simulink model "Lab4b"  (R2019b)
settings: Solver=VariableStepAuto  StartTime=0.0  StopTime=10.0  RelTol=1e-3
undefined symbols (not defined in the file): dc
libraries: dspfdesign x2, commfilt2 x1, dspstat3 x1, commsink2 x1, commsynccomp2 x1
settings Model: Creator=z3454314  LastModifiedBy=z3454314

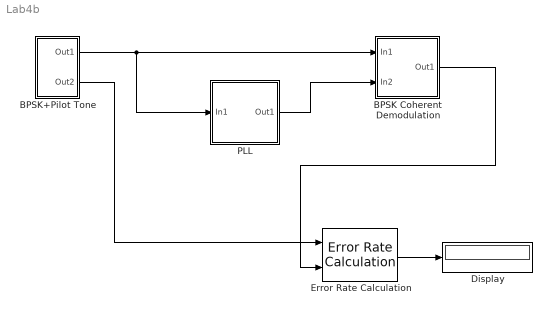
== system Lab4b ==
  BPSK Coherent Demodulation : Subsystem
  BPSK+Pilot Tone : Subsystem
  Display : Display
  Error Rate Calculation : commsink2/Error Rate Calculation  N=2  st_delay=50  cp_mode=Entire frame  subframe=[]  PMode=Port  WsName=ErrorVec  RsMode2=off  stop=off  numErr=100  maxBits=1e6
      settings: SourceProductName=Communications Toolbox
  PLL : Subsystem
  wires:
  Error Rate Calculation/1 -> Display/1
  BPSK+Pilot Tone/2(Out2) -> Error Rate Calculation/1
  BPSK Coherent Demodulation/1(Out1) -> Error Rate Calculation/2
  PLL/1(Out1) -> BPSK Coherent Demodulation/2(In2)
  BPSK+Pilot Tone/1(Out1) -> BPSK Coherent Demodulation/1(In1), PLL/1(In1)

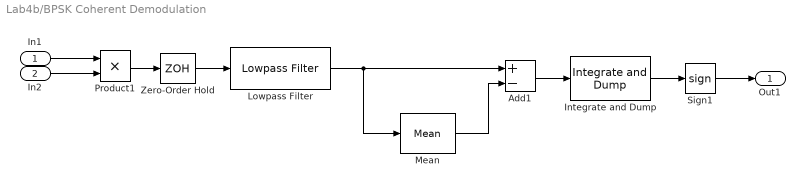
== system Lab4b/BPSK Coherent Demodulation ==
  In1 : Inport
  In2 : Inport  Port=2
  Add1 : Sum  Inputs=+-
  Integrate and Dump : commfilt2/Integrate and Dump  obssamples=1000  offsetsamples=23  nodump=off  roundingMode=Floor  overflowMode=off  outputDataTypeStr=Inherit: Same as accumulator  outputLastDataTypeStr=Inherit: Same as accumulator
      settings: SourceProductName=Communications Toolbox
  Lowpass Filter : dspfdesign/Lowpass Filter  FilterType=FIR  DesignForMinimumOrder=on  FilterOrder=50  PassbandFrequency=6e3  StopbandFrequency=10e3  PassbandRipple=0.1  StopbandAttenuation=80  InheritSampleRate=on  SampleRate=44100  SimulateUsing=Interpreted execution  roundingMode=Floor  coeffsDataTypeStr=fixdt(1,16)
  Mean : dspstat3/Mean  run=on  reset_popup=None  directionMode=Each column  dimension=1  roiEnable=off  roiType=Rectangles  roiPortion=Entire ROI  roiOutput=Individual statistics for each ROI  roiFlag=off  roundingMode=Floor  overflowMode=off  outputDataTypeStr=Inherit: Same as accumulator  outputMin=[]  outputMax=[]  outputLastDataTypeStr=Inherit: Same as accumulator
  Product1 : Product
  Sign1 : Signum
  Zero-Order Hold : ZeroOrderHold  SampleTime=1/500e3
  Out1 : Outport
  wires:
  Mean/1 -> Add1/2
  Zero-Order Hold/1 -> Lowpass Filter/1
  Lowpass Filter/1 -> Mean/1, Add1/1
  In1/1 -> Product1/1
  Integrate and Dump/1 -> Sign1/1
  Product1/1 -> Zero-Order Hold/1
  Sign1/1 -> Out1/1
  Add1/1 -> Integrate and Dump/1
  In2/1 -> Product1/2

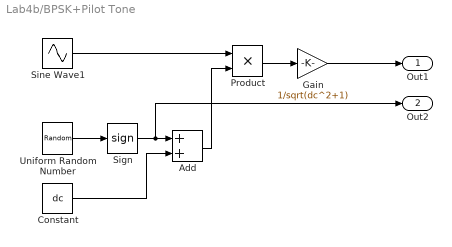
== system Lab4b/BPSK+Pilot Tone ==
  Add : Sum
  Constant : Constant  Value=dc
  Gain : Gain  Gain=1/sqrt(dc^2+1)
  Product : Product
  Sign : Signum
  Sine Wave1 : Sin  Frequency=8020*2*pi  SampleTime=0
  Uniform Random Number : UniformRandomNumber  SampleTime=1/500
  Out1 : Outport
  Out2 : Outport  Port=2
  wires:
  Constant/1 -> Add/2
  Sine Wave1/1 -> Product/1
  Gain/1 -> Out1/1
  Product/1 -> Gain/1
  Sign/1 -> Out2/1, Add/1
  Uniform Random Number/1 -> Sign/1
  Add/1 -> Product/2

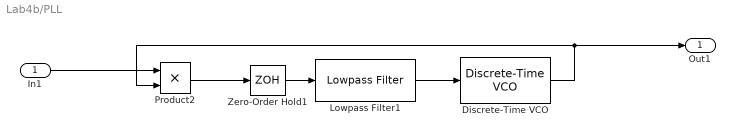
== system Lab4b/PLL ==
  In1 : Inport
  Discrete-Time VCO : commsynccomp2/Discrete-Time VCO  Ac=1  Fc=8000  Kc=100  Ph=0  ts=1/500e3
      settings: SourceProductName=Communications Toolbox  SourceProductBaseCode=CM
  Lowpass Filter1 : dspfdesign/Lowpass Filter  FilterType=FIR  DesignForMinimumOrder=on  FilterOrder=50  PassbandFrequency=5e3  StopbandFrequency=10e3  PassbandRipple=0.1  StopbandAttenuation=80  InheritSampleRate=on  SampleRate=500e3  SimulateUsing=Interpreted execution  roundingMode=Floor  coeffsDataTypeStr=fixdt(1,16)
  Product2 : Product
  Zero-Order Hold1 : ZeroOrderHold  SampleTime=1/500e3
  Out1 : Outport
  wires:
  Product2/1 -> Zero-Order Hold1/1
  Lowpass Filter1/1 -> Discrete-Time VCO/1
  Zero-Order Hold1/1 -> Lowpass Filter1/1
  Discrete-Time VCO/1 -> Out1/1, Product2/2
  In1/1 -> Product2/1
